simulink model "tank_2punkt"  (R2018b)
settings: Solver=VariableStepAuto  StartTime=0.0  StopTime=10.0  RelTol=1e-3
libraries: simulink x1
settings Model: Creator=Duc  LastModifiedBy=Duc

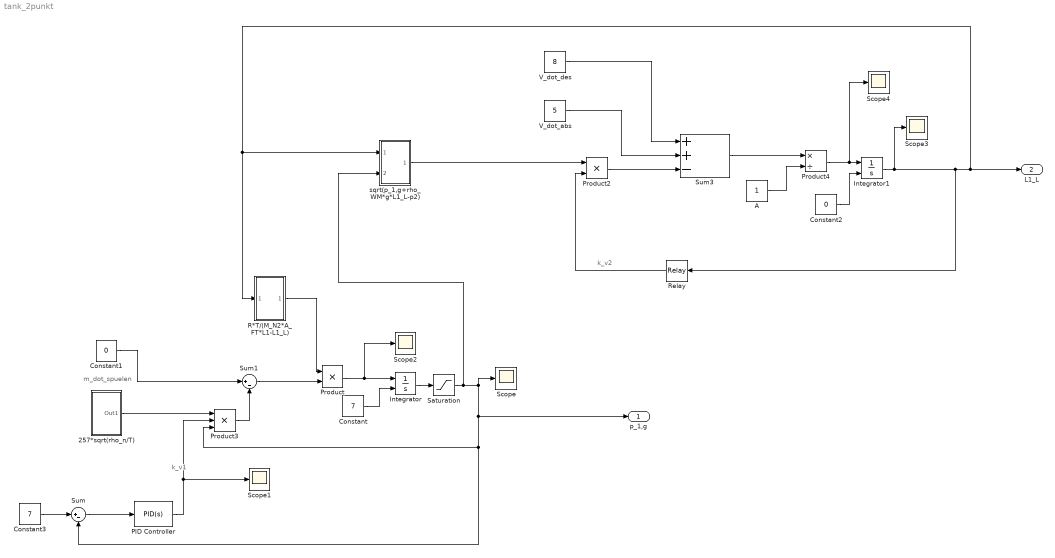
== system tank_2punkt ==
  note: k_v2
  note: m_dot_spuelen
  note: k_v1
  257*sqrt(rho_n/T) : Subsystem
  A : Constant
  Constant : Constant  Value=7
  Constant1 : Constant  Value=0
  Constant2 : Constant  Value=0
  Constant3 : Constant  Value=7
  Integrator : Integrator  InitialConditionSource=external  LowerSaturationLimit=0
  Integrator1 : Integrator  InitialConditionSource=external  LowerSaturationLimit=0
  PID Controller : simulink/Continuous/PID Controller  Controller=PID  Form=Parallel  TimeDomain=Continuous-time  SampleTime=-1  IntegratorMethod=Forward Euler  FilterMethod=Forward Euler  ControllerParametersSource=internal  P=-2  I=0  D=0  UseFilter=on  N=100  TunerSelectOption=Transfer Function Based (PID Tuner App)  InitialConditionSource=internal  InitialConditionForIntegrator=0  InitialConditionForFilter=0  DifferentiatorICPrevScaledInput=0  ExternalReset=none  TrackingMode=off  Kt=1  LimitOutput=on  UpperSaturationLimit=200  LowerSaturationLimit=0  LinearizeAsGain=on  AntiWindupMode=none  Kb=1  POutMin=[]  POutMax=[]  IOutMin=[]  IOutMax=[]  DOutMin=[]  DOutMax=[]  NOutMin=[]  NOutMax=[]  SumOutMin=[]  SumOutMax=[]  SaturationOutMin=[]  SaturationOutMax=[]  PParamMin=[]  PParamMax=[]  IParamMin=[]  IParamMax=[]  DParamMin=[]  DParamMax=[]  NParamMin=[]  NParamMax=[]  KbParamMin=[]  KbParamMax=[]  KtParamMin=[]  KtParamMax=[]  KbOutMin=[]  KbOutMax=[]  KtOutMin=[]  KtOutMax=[]  IntegratorOutMin=[]  IntegratorOutMax=[]  FilterOutMin=[]  FilterOutMax=[]  SumI1OutMin=[]  SumI1OutMax=[]  SumI2OutMin=[]  SumI2OutMax=[]  SumI3OutMin=[]  SumI3OutMax=[]  SumI4OutMin=[]  SumI4OutMax=[]  SumDOutMin=[]  SumDOutMax=[]  DifferentiatorOutMin=[]  DifferentiatorOutMax=[]  FilterDiffOutCoefMin=[]  FilterDiffOutCoefMax=[]  ReciprocalOutMin=[]  ReciprocalOutMax=[]  SumDenOutMin=[]  SumDenOutMax=[]  SumNumOutMin=[]  SumNumOutMax=[]  DivideOutMin=[]  DivideOutMax=[]  IntegratorContinuousStateAttributes=''  IntegratorStateMustResolveToSignalObject=off  IntegratorRTWStateStorageClass=Auto  FilterContinuousStateAttributes=''  FilterStateMustResolveToSignalObject=off  FilterRTWStateStorageClass=Auto  ParallelPVariant=InternalParameters  IdealPVariant=Disabled  IVariant=InternalParameters  DVariant=InternalParameters  IntegratorVariant=Continuous  SatVariant=Enabled  AWVariant=Passthrough  PCopyVariant=Disabled  TRVariant=Disabled  FdbkBlocksVariant=Forward  IdealPFdbkVariant=Disabled  SatFdbkVariant=Disabled  DerivativeFilterVariant=ContFilter  NVariant=InternalParameters  NCopyVariant=Disabled  FilterICVariant=InternalICsFilter  IntegratorICVariant=InternalICs  ExternalResetVariant=Disabled  TRSumVariant=Passthrough  SumFdbkVariant=Disabled  SumVariant=Sum_PID
  Product : Product
  Product2 : Product
  Product3 : Product  Inputs=3
  Product4 : Product  Inputs=*/
  R*T/(M_N2*A_FT*L1-L1_L) : Subsystem
  Relay : Relay  OnSwitchValue=15  OffSwitchValue=5  OnOutputValue=20
  Saturation : Saturate  UpperLimit=inf  LowerLimit=0
  Scope{,1..4} (5 alike) : Scope
  Sum : Sum  Inputs=|+-
  Sum1 : Sum  Inputs=|+-
  Sum3 : Sum  Inputs=++-
  V_dot_abs : Constant  Value=5
  V_dot_des : Constant  Value=8
  sqrt(p_1,g+rho_WM*g*L1_L-p2) : Subsystem
  p_1,g : Outport
  L1_L : Outport  Port=2
  wires:
  Sum1/1 -> Product/2
  Product3/1 -> Sum1/2
  Constant3/1 -> Sum/1
  Constant1/1 -> Sum1/1
  PID Controller/1 -> Scope1/1, Product3/2
  257*sqrt(rho_n/T)/1(Out1) -> Product3/1
  Sum/1 -> PID Controller/1
  Integrator/1 -> Saturation/1
  Constant/1 -> Integrator/2
  Product/1 -> Scope2/1, Integrator/1
  Integrator1/1 -> Relay/1, R*T/(M_N2*A_FT*L1-L1_L)/1(In1), sqrt(p_1,g+rho_WM*g*L1_L-p2)/1(In1), L1_L/1, Scope3/1
  R*T/(M_N2*A_FT*L1-L1_L)/1(Out1) -> Product/1
  Relay/1 -> Product2/2
  Product2/1 -> Sum3/3
  Sum3/1 -> Product4/1
  V_dot_abs/1 -> Sum3/2
  V_dot_des/1 -> Sum3/1
  A/1 -> Product4/2
  Product4/1 -> Scope4/1, Integrator1/1
  Constant2/1 -> Integrator1/2
  sqrt(p_1,g+rho_WM*g*L1_L-p2)/1(Out1) -> Product2/1
  Saturation/1 -> sqrt(p_1,g+rho_WM*g*L1_L-p2)/2(In2), Scope/1, Product3/3, Sum/2, p_1,g/1

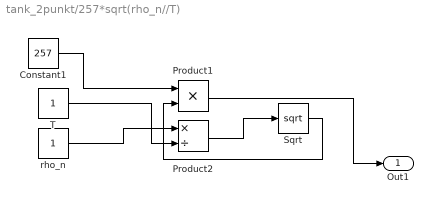
== system tank_2punkt/257*sqrt(rho_n//T) ==
  Constant1 : Constant  Value=257
  Product1 : Product
  Product2 : Product  Inputs=*/
  Sqrt : Sqrt  SaturateOnIntegerOverflow=on
  T : Constant
  rho_n : Constant
  Out1 : Outport
  wires:
  Product2/1 -> Sqrt/1
  Product1/1 -> Out1/1
  Constant1/1 -> Product1/1
  T/1 -> Product2/2
  rho_n/1 -> Product2/1
  Sqrt/1 -> Product1/2

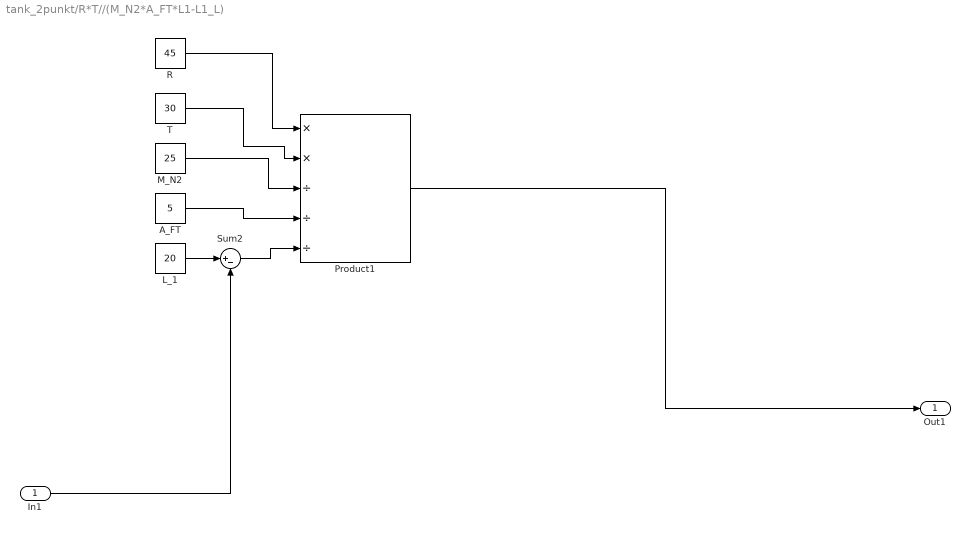
== system tank_2punkt/R*T//(M_N2*A_FT*L1-L1_L) ==
  In1 : Inport
  A_FT : Constant  Value=5
  L_1 : Constant  Value=20
  M_N2 : Constant  Value=25
  Product1 : Product  Inputs=**///
  R : Constant  Value=45
  Sum2 : Sum  Inputs=|+-
  T : Constant  Value=30
  Out1 : Outport
  wires:
  A_FT/1 -> Product1/4
  Product1/1 -> Out1/1
  T/1 -> Product1/2
  R/1 -> Product1/1
  L_1/1 -> Sum2/1
  Sum2/1 -> Product1/5
  In1/1 -> Sum2/2
  M_N2/1 -> Product1/3

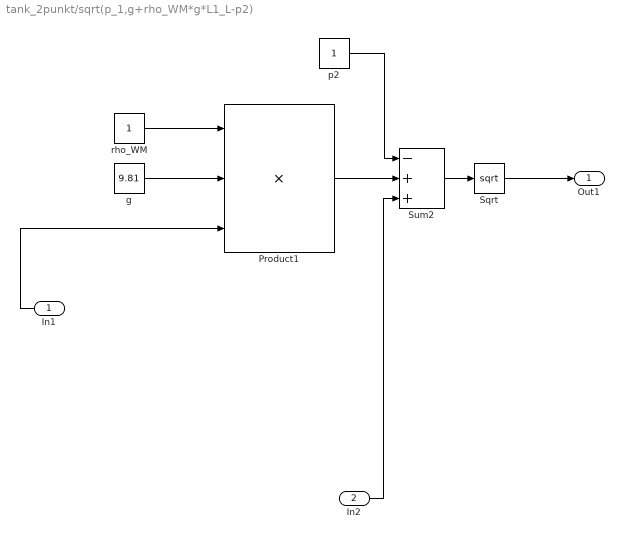
== system tank_2punkt/sqrt(p_1,g+rho_WM*g*L1_L-p2) ==
  In1 : Inport
  In2 : Inport  Port=2
  Product1 : Product  Inputs=3
  Sqrt : Sqrt  SaturateOnIntegerOverflow=on
  Sum2 : Sum  Inputs=-++
  g : Constant  Value=9.81
  p2 : Constant
  rho_WM : Constant
  Out1 : Outport
  wires:
  rho_WM/1 -> Product1/1
  Product1/1 -> Sum2/2
  g/1 -> Product1/2
  In1/1 -> Product1/3
  Sum2/1 -> Sqrt/1
  Sqrt/1 -> Out1/1
  p2/1 -> Sum2/1
  In2/1 -> Sum2/3
